simulink model "MOBATSim_AutoTesting"  (R2020b)
settings: Solver=VariableStepAuto  StartTime=0.0  StopTime=20  FixedStep=0.01  RelTol=1e-3
undefined symbols (not defined in the file or in its folder): default_spacing, FI_distance, FI_speed, max_ac, meters, min_ac, SafeDistance, Sim_Ts, simSpeed, time_gap, Ts, v_set, Vehicle1, Vehicle10, Vehicle2, Vehicle3, Vehicle4, Vehicle5, Vehicle6, Vehicle7, Vehicle8, Vehicle9, verr_gain, vx_gain, xerr_gain
libraries: simulink x21, pid_lib x11, mpcadaslib x1
(part 1 of 4)
settings Model: Creator=Mustafa  LastModifiedBy=62783
settings SolverCC: AutoInsertRateTranBlk=on  InsertRTBMode=Always  MinimalZcImpactIntegration=on
settings DataIOCC: ReturnWorkspaceOutputs=off
settings DebuggingCC: AlgebraicLoopMsg=error  ArithmeticOperatorsInVariantConditions=warning
settings SFSimCC: SimUseLocalCustomCode=off  CustomCodeUndefinedFunction=UseInterfaceOnly
settings RTWCC: RTWUseLocalCustomCode=off
settings CodeAppCC: StateflowObjectComments=on

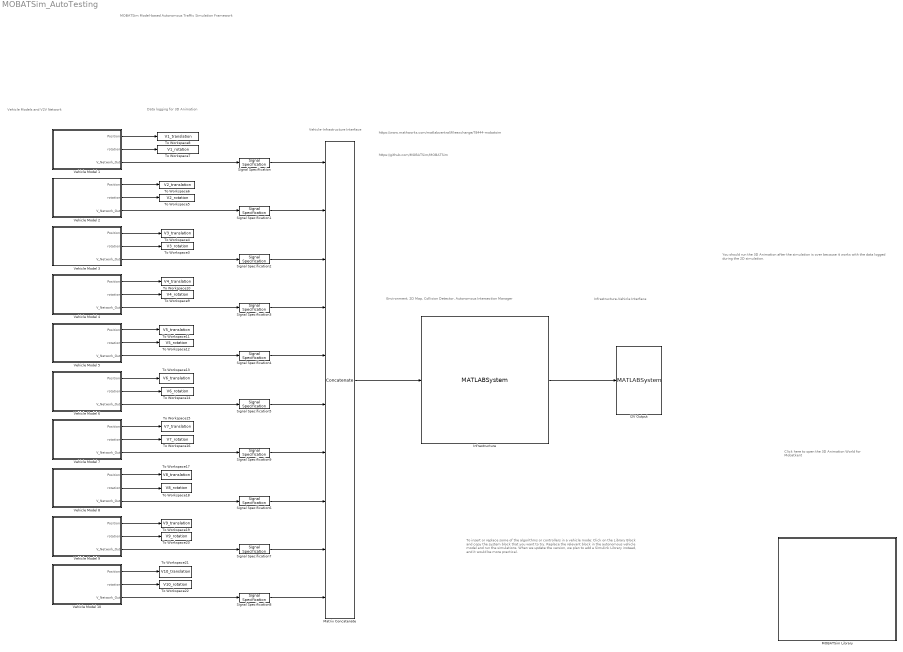
== system MOBATSim_AutoTesting ==
  note: https://www.mathworks.com/matlabcentral/fileexchange/78444-mobatsim
  note: https://github.com/MOBATSim/MOBATSim
  note: To insert or replace some of the algorithms
      | or controllers in a vehicle mode:
      | Click on the Library Block and copy the system block that you want to try.
      | Replace the relevant block in the autonomous vehicle model and run the simulations.
      | When we update the version, we plan to add a Simulink Library instead, and it would be more practical.
  note: MOBATSim
      | Model-based Autonomous Traffic Simulation Framework
  note: You should run the 3D Animation after the simulation is over because it works with the data logged during the 2D simulation.
  note: Click here to open the 3D Animation World for Mobatkent
  note: Infrastructure-Vehicle Interface
  note: Data logging for 3D Animation
  note: Vehicle Models and V2V Network
  note: Environment, 2D Map, Collision Detector, Autonomous Intersection Manager
  note: Vehicle-Infrastructure Interface
  I2V Output : MATLABSystem  System=I2V  SimulateUsing=Interpreted execution
      mask Type: I2V
      mask Display:
      | image('I2V.png');
      | port_label('input',1,'Flags');
  Infrastructure : MATLABSystem  Description=An instance of the Map.m Class is created.  System=Infrastructure  SimulateUsing=Interpreted execution
      mask Type: Infrastructure
      mask Display:
      | image('logo_small.png');
      | port_label('input',1,'V2Idata');
      | port_label('output',1,'mergedBrakingFlagArrays');
  MOBATSim Library : Subsystem
      mask Display: image('$imagefile'); % Use "Edit Image" on toolstrip to change.
  Matrix Concatenate : Concatenate  NumInputs=10  Mode=Multidimensional array
  Signal Specification{,1..9} (10 alike) : SignalSpecification  Dimensions=[1 2]
  To Workspace10 : ToWorkspace  VariableName=V4_translation  SaveFormat=Timeseries  SampleTime=-1
  To Workspace11 : ToWorkspace  VariableName=V5_translation  SaveFormat=Timeseries  SampleTime=-1
  To Workspace12 : ToWorkspace  VariableName=V5_rotation  SaveFormat=Timeseries  SampleTime=-1
  To Workspace13 : ToWorkspace  VariableName=V6_translation  SaveFormat=Timeseries  SampleTime=-1
  To Workspace14 : ToWorkspace  VariableName=V6_rotation  SaveFormat=Timeseries  SampleTime=-1
  To Workspace15 : ToWorkspace  VariableName=V7_translation  SaveFormat=Timeseries  SampleTime=-1
  To Workspace16 : ToWorkspace  VariableName=V7_rotation  SaveFormat=Timeseries  SampleTime=-1
  To Workspace17 : ToWorkspace  VariableName=V8_translation  SaveFormat=Timeseries  SampleTime=-1
  To Workspace18 : ToWorkspace  VariableName=V8_rotation  SaveFormat=Timeseries  SampleTime=-1
  To Workspace19 : ToWorkspace  VariableName=V9_translation  SaveFormat=Timeseries  SampleTime=-1
  To Workspace20 : ToWorkspace  VariableName=V9_rotation  SaveFormat=Timeseries  SampleTime=-1
  To Workspace21 : ToWorkspace  VariableName=V10_translation  SaveFormat=Timeseries  SampleTime=-1
  To Workspace22 : ToWorkspace  VariableName=V10_rotation  SaveFormat=Timeseries  SampleTime=-1
  To Workspace3 : ToWorkspace  VariableName=V3_rotation  SaveFormat=Timeseries  SampleTime=-1
  To Workspace4 : ToWorkspace  VariableName=V3_translation  SaveFormat=Timeseries  SampleTime=-1
  To Workspace5 : ToWorkspace  VariableName=V2_rotation  SaveFormat=Timeseries  SampleTime=-1
  To Workspace6 : ToWorkspace  VariableName=V2_translation  SaveFormat=Timeseries  SampleTime=-1
  To Workspace7 : ToWorkspace  VariableName=V1_rotation  SaveFormat=Timeseries  SampleTime=-1
  To Workspace8 : ToWorkspace  VariableName=V1_translation  SaveFormat=Timeseries  SampleTime=-1
  To Workspace9 : ToWorkspace  VariableName=V4_rotation  SaveFormat=Timeseries  SampleTime=-1
  Vehicle Model 1 : Subsystem  Description=Tag: Autonomous Vehicle Model  SystemSampleTime=0.01  mask{Pos=Vehicle1.dynamics.position, Vehicle_id=[1], SpeedScale=1/simSpeed, maxSpeed=Vehicle1.dynamics.maxSpeed, MinDeceleration=Vehicle1.dynamics.minDeceleration, FI_distance=FI_distance, FI_speed=FI_speed, meters=SafeDistance}
      mask prompts: Pos "Initial Position"; FI_distance "FI_Distance_Sensor"; meters "SafeDistance"
      mask TypeOptions Pos: initial position/Value
      mask TypeOptions Vehicle_id: MATLAB System2/Vehicle_id
      mask TypeOptions SpeedScale: scale the movement/Gain
      mask TypeOptions maxSpeed: Longitudinal Speed Control/Platoon Controller/Saturation3/UpperLimit
      mask TypeOptions MinDeceleration: Longitudinal Speed Control/Acceleration Command/Emergency Brake/Value
      mask TypeOptions FI_distance: Fault Injection Percentage/Value
      mask TypeOptions FI_speed: Longitudinal Speed Control/FI Freeze/Constant/Value
      mask TypeOptions meters: Longitudinal Speed Control/Platoon Controller/Constant/Value
      mask DialogControl DescTextVar Prompt: Autonomous Vehicle Model defined as a system, press the arrow on the lower left corner to see the subsystems. The initial parameters below should be taken from the base workspace but you can edit them anyway you like.
      mask Display: image('$imagefile'); % Use "Edit Image" on toolstrip to change.
  Vehicle Model 10 : Subsystem  Description=Tag: Autonomous Vehicle Model  SystemSampleTime=0.01  mask{Pos=Vehicle10.dynamics.position, Vehicle_id=[10], SpeedScale=1/simSpeed, maxSpeed=Vehicle10.dynamics.maxSpeed, MinDeceleration=Vehicle10.dynamics.minDeceleration, FI_distance=FI_distance, FI_speed=FI_speed, meters=SafeDistance}
      mask prompts: Pos "Initial Position"; FI_distance "FI_Distance_Sensor"; meters "SafeDistance"
      mask TypeOptions Pos: initial position/Value
      mask TypeOptions Vehicle_id: MATLAB System2/Vehicle_id
      mask TypeOptions SpeedScale: scale the movement/Gain
      mask TypeOptions maxSpeed: Longitudinal Speed Control/Platoon Controller/Saturation3/UpperLimit
      mask TypeOptions MinDeceleration: Longitudinal Speed Control/Acceleration Command/Emergency Brake/Value
      mask TypeOptions FI_distance: Fault Injection Percentage/Value
      mask TypeOptions FI_speed: Longitudinal Speed Control/FI Freeze/Constant/Value
      mask TypeOptions meters: Longitudinal Speed Control/Platoon Controller/Constant/Value
      mask DialogControl DescTextVar Prompt: Autonomous Vehicle Model defined as a system, press the arrow on the lower left corner to see the subsystems. The initial parameters below should be taken from the base workspace but you can edit them anyway you like.
      mask Display: image('redcar.png'); % Use "Edit Image" on toolstrip to change.
  Vehicle Model 2 : Subsystem  Description=Tag: Autonomous Vehicle Model  SystemSampleTime=0.01  mask{Pos=Vehicle2.dynamics.position, Vehicle_id=[2], SpeedScale=1/simSpeed, maxSpeed=Vehicle2.dynamics.maxSpeed, MinDeceleration=Vehicle2.dynamics.minDeceleration, FI_distance=FI_distance, FI_speed=FI_speed, meters=SafeDistance}
      mask prompts: Pos "Initial Position"; FI_distance "FI_Distance_Sensor"; meters "SafeDistance"
      mask TypeOptions Pos: initial position/Value
      mask TypeOptions Vehicle_id: MATLAB System2/Vehicle_id
      mask TypeOptions SpeedScale: scale the movement/Gain
      mask TypeOptions maxSpeed: Longitudinal Speed Control/Platoon Controller/Saturation3/UpperLimit
      mask TypeOptions MinDeceleration: Longitudinal Speed Control/Acceleration Command/Emergency Brake/Value
      mask TypeOptions FI_distance: Fault Injection Percentage/Value
      mask TypeOptions FI_speed: Longitudinal Speed Control/FI Freeze/Constant/Value
      mask TypeOptions meters: Longitudinal Speed Control/Platoon Controller/Constant/Value
      mask DialogControl DescTextVar Prompt: Autonomous Vehicle Model defined as a system, press the arrow on the lower left corner to see the subsystems. The initial parameters below should be taken from the base workspace but you can edit them anyway you like.
      mask Display: image('$imagefile'); % Use "Edit Image" on toolstrip to change.
  Vehicle Model 3 : Subsystem  Description=Tag: Autonomous Vehicle Model  SystemSampleTime=0.01  mask{Pos=Vehicle3.dynamics.position, Vehicle_id=[3], SpeedScale=1/simSpeed, maxSpeed=Vehicle3.dynamics.maxSpeed, MinDeceleration=Vehicle3.dynamics.minDeceleration, FI_distance=FI_distance, FI_speed=FI_speed, meters=SafeDistance}
      mask prompts: Pos "Initial Position"; FI_distance "FI_Distance_Sensor"; meters "SafeDistance"
      mask TypeOptions Pos: initial position/Value
      mask TypeOptions Vehicle_id: MATLAB System2/Vehicle_id
      mask TypeOptions SpeedScale: scale the movement/Gain
      mask TypeOptions maxSpeed: Longitudinal Speed Control/Platoon Controller/Saturation3/UpperLimit
      mask TypeOptions MinDeceleration: Longitudinal Speed Control/Acceleration Command/Emergency Brake/Value
      mask TypeOptions FI_distance: Fault Injection Percentage/Value
      mask TypeOptions FI_speed: Longitudinal Speed Control/FI Freeze/Constant/Value
      mask TypeOptions meters: Longitudinal Speed Control/Platoon Controller/Constant/Value
      mask DialogControl DescTextVar Prompt: Autonomous Vehicle Model defined as a system, press the arrow on the lower left corner to see the subsystems. The initial parameters below should be taken from the base workspace but you can edit them anyway you like.
      mask Display: image('$imagefile'); % Use "Edit Image" on toolstrip to change.
  Vehicle Model 4 : Subsystem  Description=Tag: Autonomous Vehicle Model  SystemSampleTime=0.01  mask{Pos=Vehicle4.dynamics.position, Vehicle_id=[4], SpeedScale=1/simSpeed, maxSpeed=Vehicle4.dynamics.maxSpeed, MinDeceleration=Vehicle4.dynamics.minDeceleration, FI_distance=FI_distance, FI_speed=FI_speed, meters=SafeDistance}
      mask prompts: Pos "Initial Position"; FI_distance "FI_Distance_Sensor"; meters "SafeDistance"
      mask TypeOptions Pos: initial position/Value
      mask TypeOptions Vehicle_id: MATLAB System2/Vehicle_id
      mask TypeOptions SpeedScale: scale the movement/Gain
      mask TypeOptions maxSpeed: Longitudinal Speed Control/Platoon Controller/Saturation3/UpperLimit
      mask TypeOptions MinDeceleration: Longitudinal Speed Control/Acceleration Command/Emergency Brake/Value
      mask TypeOptions FI_distance: Fault Injection Percentage/Value
      mask TypeOptions FI_speed: Longitudinal Speed Control/FI Freeze/Constant/Value
      mask TypeOptions meters: Longitudinal Speed Control/Platoon Controller/Constant/Value
      mask DialogControl DescTextVar Prompt: Autonomous Vehicle Model defined as a system, press the arrow on the lower left corner to see the subsystems. The initial parameters below should be taken from the base workspace but you can edit them anyway you like.
      mask Display: image('$imagefile'); % Use "Edit Image" on toolstrip to change.
  Vehicle Model 5 : Subsystem  Description=Tag: Autonomous Vehicle Model  SystemSampleTime=0.01  mask{Pos=Vehicle5.dynamics.position, Vehicle_id=[5], SpeedScale=1/simSpeed, maxSpeed=Vehicle5.dynamics.maxSpeed, MinDeceleration=Vehicle5.dynamics.minDeceleration, FI_distance=FI_distance, FI_speed=FI_speed, meters=SafeDistance}
      mask prompts: Pos "Initial Position"; FI_distance "FI_Distance_Sensor"; meters "SafeDistance"
      mask TypeOptions Pos: initial position/Value
      mask TypeOptions Vehicle_id: MATLAB System2/Vehicle_id
      mask TypeOptions SpeedScale: scale the movement/Gain
      mask TypeOptions maxSpeed: Longitudinal Speed Control/Platoon Controller/Saturation3/UpperLimit
      mask TypeOptions MinDeceleration: Longitudinal Speed Control/Acceleration Command/Emergency Brake/Value
      mask TypeOptions FI_distance: Fault Injection Percentage/Value
      mask TypeOptions FI_speed: Longitudinal Speed Control/FI Freeze/Constant/Value
      mask TypeOptions meters: Longitudinal Speed Control/Platoon Controller/Constant/Value
      mask DialogControl DescTextVar Prompt: Autonomous Vehicle Model defined as a system, press the arrow on the lower left corner to see the subsystems. The initial parameters below should be taken from the base workspace but you can edit them anyway you like.
      mask Display: image('$imagefile'); % Use "Edit Image" on toolstrip to change.
  Vehicle Model 6 : Subsystem  Description=Tag: Autonomous Vehicle Model  SystemSampleTime=0.01  mask{Pos=Vehicle6.dynamics.position, Vehicle_id=[6], SpeedScale=1/simSpeed, maxSpeed=Vehicle6.dynamics.maxSpeed, MinDeceleration=Vehicle6.dynamics.minDeceleration, FI_distance=FI_distance, FI_speed=FI_speed, meters=SafeDistance}
      mask prompts: Pos "Initial Position"; FI_distance "FI_Distance_Sensor"; meters "SafeDistance"
      mask TypeOptions Pos: initial position/Value
      mask TypeOptions Vehicle_id: MATLAB System2/Vehicle_id
      mask TypeOptions SpeedScale: scale the movement/Gain
      mask TypeOptions maxSpeed: Longitudinal Speed Control/Platoon Controller/Saturation3/UpperLimit
      mask TypeOptions MinDeceleration: Longitudinal Speed Control/Acceleration Command/Emergency Brake/Value
      mask TypeOptions FI_distance: Fault Injection Percentage/Value
      mask TypeOptions FI_speed: Longitudinal Speed Control/FI Freeze/Constant/Value
      mask TypeOptions meters: Longitudinal Speed Control/Platoon Controller/Constant/Value
      mask DialogControl DescTextVar Prompt: Autonomous Vehicle Model defined as a system, press the arrow on the lower left corner to see the subsystems. The initial parameters below should be taken from the base workspace but you can edit them anyway you like.
      mask Display: image('firetruck.png'); % Use "Edit Image" on toolstrip to change.
  Vehicle Model 7 : Subsystem  Description=Tag: Autonomous Vehicle Model  SystemSampleTime=0.01  mask{Pos=Vehicle7.dynamics.position, Vehicle_id=[7], SpeedScale=1/simSpeed, maxSpeed=Vehicle7.dynamics.maxSpeed, MinDeceleration=Vehicle7.dynamics.minDeceleration, FI_distance=FI_distance, FI_speed=FI_speed, meters=SafeDistance}
      mask prompts: Pos "Initial Position"; FI_distance "FI_Distance_Sensor"; meters "SafeDistance"
      mask TypeOptions Pos: initial position/Value
      mask TypeOptions Vehicle_id: MATLAB System2/Vehicle_id
      mask TypeOptions SpeedScale: scale the movement/Gain
      mask TypeOptions maxSpeed: Longitudinal Speed Control/Platoon Controller/Saturation3/UpperLimit
      mask TypeOptions MinDeceleration: Longitudinal Speed Control/Acceleration Command/Emergency Brake/Value
      mask TypeOptions FI_distance: Fault Injection Percentage/Value
      mask TypeOptions FI_speed: Longitudinal Speed Control/FI Freeze/Constant/Value
      mask TypeOptions meters: Longitudinal Speed Control/Platoon Controller/Constant/Value
      mask DialogControl DescTextVar Prompt: Autonomous Vehicle Model defined as a system, press the arrow on the lower left corner to see the subsystems. The initial parameters below should be taken from the base workspace but you can edit them anyway you like.
      mask Display: image('$imagefile'); % Use "Edit Image" on toolstrip to change.
  Vehicle Model 8 : Subsystem  Description=Tag: Autonomous Vehicle Model  SystemSampleTime=0.01  mask{Pos=Vehicle8.dynamics.position, Vehicle_id=[8], SpeedScale=1/simSpeed, maxSpeed=Vehicle8.dynamics.maxSpeed, MinDeceleration=Vehicle8.dynamics.minDeceleration, FI_distance=FI_distance, FI_speed=FI_speed, meters=SafeDistance}
      mask prompts: Pos "Initial Position"; FI_distance "FI_Distance_Sensor"; meters "SafeDistance"
      mask TypeOptions Pos: initial position/Value
      mask TypeOptions Vehicle_id: MATLAB System2/Vehicle_id
      mask TypeOptions SpeedScale: scale the movement/Gain
      mask TypeOptions maxSpeed: Longitudinal Speed Control/Platoon Controller/Saturation3/UpperLimit
      mask TypeOptions MinDeceleration: Longitudinal Speed Control/Acceleration Command/Emergency Brake/Value
      mask TypeOptions FI_distance: Fault Injection Percentage/Value
      mask TypeOptions FI_speed: Longitudinal Speed Control/FI Freeze/Constant/Value
      mask TypeOptions meters: Longitudinal Speed Control/Platoon Controller/Constant/Value
      mask DialogControl DescTextVar Prompt: Autonomous Vehicle Model defined as a system, press the arrow on the lower left corner to see the subsystems. The initial parameters below should be taken from the base workspace but you can edit them anyway you like.
      mask Display: image('$imagefile'); % Use "Edit Image" on toolstrip to change.
  Vehicle Model 9 : Subsystem  Description=Tag: Autonomous Vehicle Model  SystemSampleTime=0.01  mask{Pos=Vehicle9.dynamics.position, Vehicle_id=[9], SpeedScale=1/simSpeed, maxSpeed=Vehicle9.dynamics.maxSpeed, MinDeceleration=Vehicle9.dynamics.minDeceleration, FI_distance=FI_distance, FI_speed=FI_speed, meters=SafeDistance}
      mask prompts: Pos "Initial Position"; FI_distance "FI_Distance_Sensor"; meters "SafeDistance"
      mask TypeOptions Pos: initial position/Value
      mask TypeOptions Vehicle_id: MATLAB System2/Vehicle_id
      mask TypeOptions SpeedScale: scale the movement/Gain
      mask TypeOptions maxSpeed: Longitudinal Speed Control/Platoon Controller/Saturation3/UpperLimit
      mask TypeOptions MinDeceleration: Longitudinal Speed Control/Acceleration Command/Emergency Brake/Value
      mask TypeOptions FI_distance: Fault Injection Percentage/Value
      mask TypeOptions FI_speed: Longitudinal Speed Control/FI Freeze/Constant/Value
      mask TypeOptions meters: Longitudinal Speed Control/Platoon Controller/Constant/Value
      mask DialogControl DescTextVar Prompt: Autonomous Vehicle Model defined as a system, press the arrow on the lower left corner to see the subsystems. The initial parameters below should be taken from the base workspace but you can edit them anyway you like.
      mask Display: image('$imagefile'); % Use "Edit Image" on toolstrip to change.
  wires:
  Vehicle Model 1/1(Position) -> To Workspace8/1
  Vehicle Model 1/2(rotation) -> To Workspace7/1
  Vehicle Model 1/3(V_Network_Out) -> Signal Specification/1
  Signal Specification/1 -> Matrix Concatenate/1
  Signal Specification1/1 -> Matrix Concatenate/2
  Vehicle Model 2/2(rotation) -> To Workspace5/1
  Vehicle Model 2/1(Position) -> To Workspace6/1
  Vehicle Model 3/2(rotation) -> To Workspace3/1
  Vehicle Model 3/1(Position) -> To Workspace4/1
  Signal Specification2/1 -> Matrix Concatenate/3
  Infrastructure/1 -> I2V Output/1
  Vehicle Model 8/3(V_Network_Out) -> Signal Specification6/1
  Vehicle Model 9/3(V_Network_Out) -> Signal Specification7/1
  Vehicle Model 10/3(V_Network_Out) -> Signal Specification8/1
  Signal Specification3/1 -> Matrix Concatenate/4
  Signal Specification4/1 -> Matrix Concatenate/5
  Signal Specification5/1 -> Matrix Concatenate/6
  Signal Specification9/1 -> Matrix Concatenate/7
  Signal Specification6/1 -> Matrix Concatenate/8
  Signal Specification7/1 -> Matrix Concatenate/9
  Signal Specification8/1 -> Matrix Concatenate/10
  Vehicle Model 4/2(rotation) -> To Workspace9/1
  Vehicle Model 4/1(Position) -> To Workspace10/1
  Vehicle Model 5/1(Position) -> To Workspace11/1
  Vehicle Model 5/2(rotation) -> To Workspace12/1
  Vehicle Model 6/2(rotation) -> To Workspace14/1
  Vehicle Model 6/1(Position) -> To Workspace13/1
  Vehicle Model 7/2(rotation) -> To Workspace16/1
  Vehicle Model 7/1(Position) -> To Workspace15/1
  Vehicle Model 8/2(rotation) -> To Workspace18/1
  Vehicle Model 8/1(Position) -> To Workspace17/1
  Vehicle Model 9/2(rotation) -> To Workspace20/1
  Vehicle Model 9/1(Position) -> To Workspace19/1
  Vehicle Model 10/2(rotation) -> To Workspace22/1
  Vehicle Model 10/1(Position) -> To Workspace21/1
  Matrix Concatenate/1 -> Infrastructure/1
  Vehicle Model 2/3(V_Network_Out) -> Signal Specification1/1
  Vehicle Model 3/3(V_Network_Out) -> Signal Specification2/1
  Vehicle Model 4/3(V_Network_Out) -> Signal Specification3/1
  Vehicle Model 5/3(V_Network_Out) -> Signal Specification4/1
  Vehicle Model 6/3(V_Network_Out) -> Signal Specification5/1
  Vehicle Model 7/3(V_Network_Out) -> Signal Specification9/1

== system MOBATSim_AutoTesting/MOBATSim Library ==
  note: Different pathplanner algorithms with the same input/outputs. Some details and computational performances may differ.
  note: The ACC Classical Block from the MathWorks Example:
      | https://www.mathworks.com/help/driving/examples/adaptive-cruise-control-with-sensor-fusion.html
  note: Path Planners - MATLAB System Blocks
  note: Platoon Controllers - Subsystem Blocks
  note: Platoon controller-PID with a safe distance controller for safely following the
      | leading vehicle. Most vehicles have this block because it is simple and fast
      | in terms of execution time. Can be tuned.
  note: Standard MPC - Adaptive Cruise Control Block. Safest option but computationally
      | expensive. Tradeoff between safety and computational performance depends on
      | the prediction horizon variable.
  ACC Classical : Subsystem  Commented=on  TreatAsAtomicUnit=on  VariantControl=controller_type == 1
      settings: RTWFileNameOpts=Use function name
  Adaptive Cruise Control System : mpcadaslib/Adaptive Cruise Control System  Commented=on  EgoModel=tf(1,[0.5,1,0])  InitialEgoVelocity=20  DefaultSpacing=10  MaxVelocity=50  MinAcceleration=-3  amin_ext=off  MaxAcceleration=2  amax_ext=off  Ts=0.1  PredictionHorizon=30  ControllerBehavior=0.5  suboptimal=off  maxiter=10  datatypeopt=double  optmode=off  trackmode=off
  Path Planner - AStar : MATLABSystem  Commented=on  System=VehiclePathPlanner  Vehicle_id=[]  SimulateUsing=Code generation
      mask Type: VehiclePathPlanner
      mask Display:
      | disp('VehiclePathPlanner');
      | port_label('input',1,'OtherVehiclesFutureData');
      | port_label('output',1,'FuturePlan');
      | port_label('output',2,'waypointReached');
  Path Planner - DStar : MATLABSystem  Commented=on  System=VehiclePathPlanner_DStarExtraLight  Vehicle_id=[]  SimulateUsing=Code generation
      mask Type: VehiclePathPlanner_DStarExtraLight
      mask Display:
      | disp('VehiclePathPlanner_DStarExtraLight');
      | port_label('input',1,'OtherVehiclesFutureData');
      | port_label('output',1,'FuturePlan');
      | port_label('output',2,'waypointReached');
  Path Planner - Shortest : MATLABSystem  Commented=on  System=VehiclePathPlanner_shortestPathFinder  Vehicle_id=[]  SimulateUsing=Code generation
      mask Type: VehiclePathPlanner_shortestPathFinder
      mask Display:
      | disp('VehiclePathPlanner_shortestPathFinder');
      | port_label('input',1,'OtherVehiclesFutureData');
      | port_label('output',1,'FuturePlan');
      | port_label('output',2,'waypointReached');
  Platoon Controller - PID : Subsystem  Commented=on

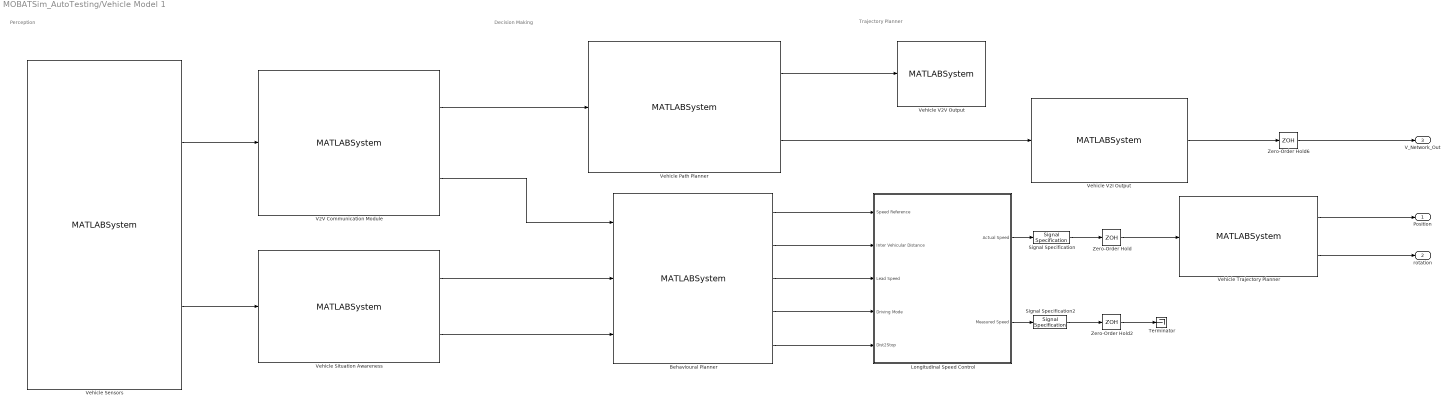
== system MOBATSim_AutoTesting/Vehicle Model 1 ==
  note: Trajectory Planner
  note: Perception
  note: Decision Making
  Behavioural Planner : MATLABSystem  System=VehicleDrivingMode  Vehicle_id=Vehicle_id  SimulateUsing=Interpreted execution
      mask Type: VehicleDrivingMode
      mask Display:
      | image('BehaviouralPlanner.png');
      | port_label('input',1,'LeaderSpeed');
      | port_label('input',2,'LeaderDistance');
      | port_label('input',3,'emergencyCase');
      | port_label('output',1,'SpeedReference');
      | port_label('output',2,'DistanceReference');
      | port_label('output',3,'LeadSpeed');
      | port_label('output',4,'DrivingMode');
      | port_label('output',5,'Dist2Stop');
  Longitudinal Speed Control : Subsystem
  Signal Specification : SignalSpecification  Dimensions=1
  Signal Specification2 : SignalSpecification  Dimensions=1
  Terminator : Terminator
  V2V Communication Module : MATLABSystem  System=VehicleCommunication_v2v  Vehicle_id=Vehicle_id  SimulateUsing=Interpreted execution
      mask Type: VehicleCommunication_v2v
      mask Display:
      | image('V2V.png');
      | port_label('input',1,'CommunicationID');
      | port_label('output',1,'OtherVehiclesFutureData');
      | port_label('output',2,'LeaderSpeed');
  Vehicle Path Planner : MATLABSystem  System=VehiclePathPlanner  Vehicle_id=Vehicle_id  SimulateUsing=Interpreted execution
      mask Type: VehiclePathPlanner
      mask Display:
      | image('PathPlanner.png');
      | port_label('input',1,'OtherVehiclesFutureData');
      | port_label('output',1,'FuturePlan');
      | port_label('output',2,'waypointReached');
  Vehicle Sensors : MATLABSystem  System=VehicleSensors  Vehicle_id=Vehicle_id  Tsample=Sim_Ts  OffsetTime=0  SimulateUsing=Interpreted execution
      mask Type: VehicleSensors
      mask Display:
      | image('sensor.png');
      | port_label('output',1,'V2VcommIDs');
      | port_label('output',2,'ObjectinFront');
  Vehicle Situation Awareness : MATLABSystem  System=VehicleSituationAwareness  Vehicle_id=Vehicle_id  SimulateUsing=Interpreted execution
      mask Type: VehicleSituationAwareness
      mask Display:
      | image('situationAwareness.png');
      | port_label('input',1,'FrontSensorData');
      | port_label('output',1,'leaderDistance');
      | port_label('output',2,'emergencyCase');
  Vehicle Trajectory Planner : MATLABSystem  System=VehicleKinematics  Vehicle_id=Vehicle_id  SimulateUsing=Interpreted execution
      mask Type: VehicleKinematics
      mask Display:
      | image('Vehicle.png');
      | port_label('input',1,'speed');
      | port_label('output',1,'position');
      | port_label('output',2,'rotation');
  Vehicle V2I Output : MATLABSystem  System=VehicleV2I_Out  Vehicle_id=Vehicle_id  SimulateUsing=Interpreted execution
      mask Type: VehicleV2I_Out
      mask Display:
      | image('V2I.png');
      | port_label('input',1,'waypointReached');
      | port_label('output',1,'V2Idata');
  Vehicle V2V Output : MATLABSystem  System=VehicleNetwork_Out  Vehicle_id=Vehicle_id  SimulateUsing=Interpreted execution
      mask Type: VehicleNetwork_Out
      mask Display:
      | image('V2V.png');
      | port_label('input',1,'FuturePlan');
  Zero-Order Hold : ZeroOrderHold  SampleTime=Sim_Ts
  Zero-Order Hold2 : ZeroOrderHold  SampleTime=Sim_Ts
  Zero-Order Hold6 : ZeroOrderHold  SampleTime=Sim_Ts
  Position : Outport  VectorParamsAs1DForOutWhenUnconnected=off
  rotation : Outport  Port=2  VectorParamsAs1DForOutWhenUnconnected=off
  V_Network_Out : Outport  Port=3  VectorParamsAs1DForOutWhenUnconnected=off
  wires:
  Vehicle Trajectory Planner/1 -> Position/1
  Vehicle Trajectory Planner/2 -> rotation/1
  Signal Specification/1 -> Zero-Order Hold/1
  Zero-Order Hold/1 -> Vehicle Trajectory Planner/1
  Signal Specification2/1 -> Zero-Order Hold2/1
  Longitudinal Speed Control/1(Actual Speed) -> Signal Specification/1
  Vehicle V2I Output/1 -> Zero-Order Hold6/1
  Longitudinal Speed Control/2(Measured Speed) -> Signal Specification2/1
  Zero-Order Hold2/1 -> Terminator/1
  Vehicle Sensors/2 -> Vehicle Situation Awareness/1
  Vehicle Situation Awareness/2 -> Behavioural Planner/3
  Vehicle Situation Awareness/1 -> Behavioural Planner/2
  V2V Communication Module/2 -> Behavioural Planner/1
  V2V Communication Module/1 -> Vehicle Path Planner/1
  Behavioural Planner/5 -> Longitudinal Speed Control/5(Dist2Stop)
  Behavioural Planner/4 -> Longitudinal Speed Control/4(Driving Mode)
  Behavioural Planner/3 -> Longitudinal Speed Control/3(Lead Speed)
  Behavioural Planner/2 -> Longitudinal Speed Control/2(Inter Vehicular Distance)
  Behavioural Planner/1 -> Longitudinal Speed Control/1(Speed Reference)
  Vehicle Path Planner/2 -> Vehicle V2I Output/1
  Vehicle Path Planner/1 -> Vehicle V2V Output/1
  Vehicle Sensors/1 -> V2V Communication Module/1
  Zero-Order Hold6/1 -> V_Network_Out/1

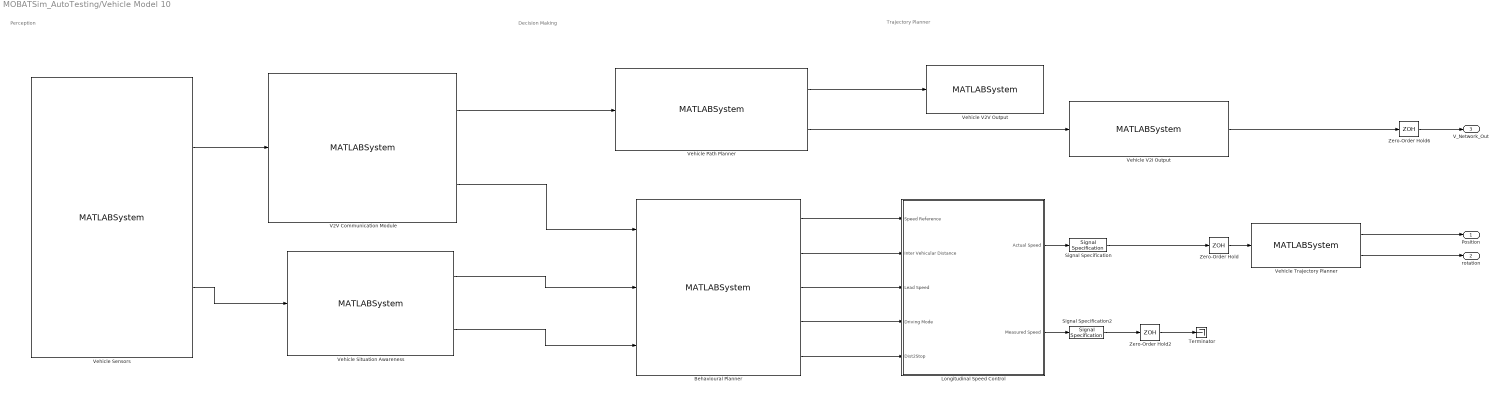
== system MOBATSim_AutoTesting/Vehicle Model 10 ==
  note: Trajectory Planner
  note: Perception
  note: Decision Making
  Behavioural Planner : MATLABSystem  System=VehicleDrivingMode  Vehicle_id=Vehicle_id  SimulateUsing=Interpreted execution
      mask Type: VehicleDrivingMode
      mask Display:
      | image('BehaviouralPlanner.png');
      | port_label('input',1,'LeaderSpeed');
      | port_label('input',2,'LeaderDistance');
      | port_label('input',3,'emergencyCase');
      | port_label('output',1,'SpeedReference');
      | port_label('output',2,'DistanceReference');
      | port_label('output',3,'LeadSpeed');
      | port_label('output',4,'DrivingMode');
      | port_label('output',5,'Dist2Stop');
  Longitudinal Speed Control : Subsystem
  Signal Specification : SignalSpecification  Dimensions=1
  Signal Specification2 : SignalSpecification  Dimensions=1
  Terminator : Terminator
  V2V Communication Module : MATLABSystem  System=VehicleCommunication_v2v  Vehicle_id=Vehicle_id  SimulateUsing=Interpreted execution
      mask Type: VehicleCommunication_v2v
      mask Display:
      | image('V2V.png');
      | port_label('input',1,'CommunicationID');
      | port_label('output',1,'OtherVehiclesFutureData');
      | port_label('output',2,'LeaderSpeed');
  Vehicle Path Planner : MATLABSystem  System=VehiclePathPlanner  Vehicle_id=Vehicle_id  SimulateUsing=Interpreted execution
      mask Type: VehiclePathPlanner
      mask Display:
      | image('PathPlanner.png');
      | port_label('input',1,'OtherVehiclesFutureData');
      | port_label('output',1,'FuturePlan');
      | port_label('output',2,'waypointReached');
  Vehicle Sensors : MATLABSystem  System=VehicleSensors  Vehicle_id=Vehicle_id  Tsample=Sim_Ts  OffsetTime=0  SimulateUsing=Interpreted execution
      mask Type: VehicleSensors
      mask Display:
      | image('sensor.png');
      | port_label('output',1,'V2VcommIDs');
      | port_label('output',2,'ObjectinFront');
  Vehicle Situation Awareness : MATLABSystem  System=VehicleSituationAwareness  Vehicle_id=Vehicle_id  SimulateUsing=Interpreted execution
      mask Type: VehicleSituationAwareness
      mask Display:
      | image('situationAwareness.png');
      | port_label('input',1,'FrontSensorData');
      | port_label('output',1,'leaderDistance');
      | port_label('output',2,'emergencyCase');
  Vehicle Trajectory Planner : MATLABSystem  System=VehicleKinematics  Vehicle_id=Vehicle_id  SimulateUsing=Interpreted execution
      mask Type: VehicleKinematics
      mask Display:
      | image('Vehicle.png');
      | port_label('input',1,'speed');
      | port_label('output',1,'position');
      | port_label('output',2,'rotation');
  Vehicle V2I Output : MATLABSystem  System=VehicleV2I_Out  Vehicle_id=Vehicle_id  SimulateUsing=Interpreted execution
      mask Type: VehicleV2I_Out
      mask Display:
      | image('V2I.png');
      | port_label('input',1,'waypointReached');
      | port_label('output',1,'V2Idata');
  Vehicle V2V Output : MATLABSystem  System=VehicleNetwork_Out  Vehicle_id=Vehicle_id  SimulateUsing=Interpreted execution
      mask Type: VehicleNetwork_Out
      mask Display:
      | image('V2V.png');
      | port_label('input',1,'FuturePlan');
  Zero-Order Hold : ZeroOrderHold  SampleTime=Sim_Ts
  Zero-Order Hold2 : ZeroOrderHold  SampleTime=Sim_Ts
  Zero-Order Hold6 : ZeroOrderHold  SampleTime=Sim_Ts
  Position : Outport  VectorParamsAs1DForOutWhenUnconnected=off
  rotation : Outport  Port=2  VectorParamsAs1DForOutWhenUnconnected=off
  V_Network_Out : Outport  Port=3  VectorParamsAs1DForOutWhenUnconnected=off
  wires:
  Vehicle Trajectory Planner/1 -> Position/1
  Vehicle Trajectory Planner/2 -> rotation/1
  Signal Specification/1 -> Zero-Order Hold/1
  Zero-Order Hold/1 -> Vehicle Trajectory Planner/1
  Signal Specification2/1 -> Zero-Order Hold2/1
  Longitudinal Speed Control/1(Actual Speed) -> Signal Specification/1
  Vehicle V2I Output/1 -> Zero-Order Hold6/1
  Longitudinal Speed Control/2(Measured Speed) -> Signal Specification2/1
  Zero-Order Hold2/1 -> Terminator/1
  Vehicle Sensors/2 -> Vehicle Situation Awareness/1
  Vehicle Situation Awareness/2 -> Behavioural Planner/3
  Vehicle Situation Awareness/1 -> Behavioural Planner/2
  V2V Communication Module/2 -> Behavioural Planner/1
  V2V Communication Module/1 -> Vehicle Path Planner/1
  Behavioural Planner/5 -> Longitudinal Speed Control/5(Dist2Stop)
  Behavioural Planner/4 -> Longitudinal Speed Control/4(Driving Mode)
  Behavioural Planner/3 -> Longitudinal Speed Control/3(Lead Speed)
  Behavioural Planner/2 -> Longitudinal Speed Control/2(Inter Vehicular Distance)
  Behavioural Planner/1 -> Longitudinal Speed Control/1(Speed Reference)
  Vehicle Path Planner/2 -> Vehicle V2I Output/1
  Vehicle Path Planner/1 -> Vehicle V2V Output/1
  Vehicle Sensors/1 -> V2V Communication Module/1
  Zero-Order Hold6/1 -> V_Network_Out/1

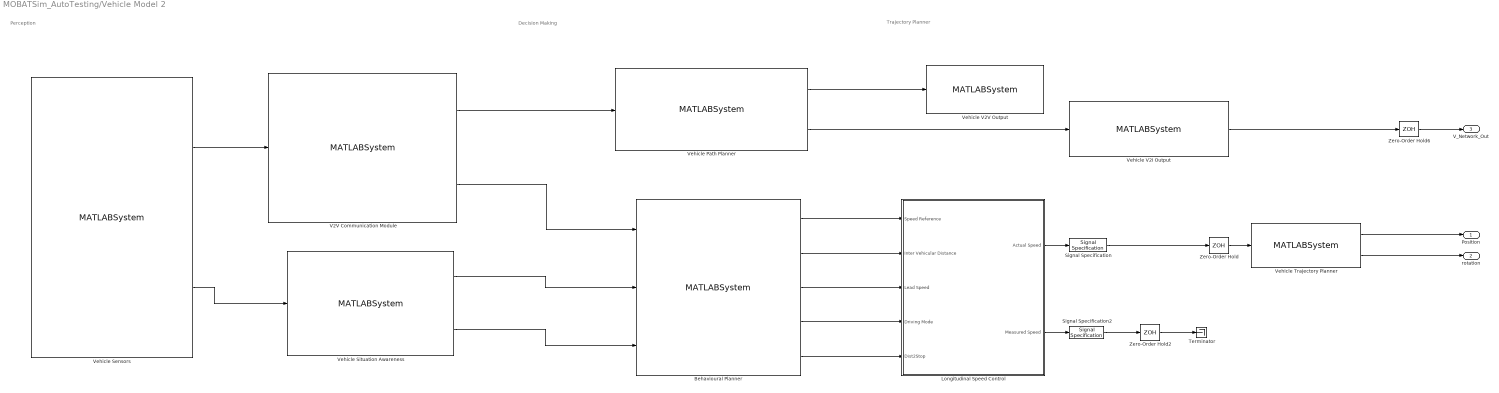
== system MOBATSim_AutoTesting/Vehicle Model 2 ==
  note: Trajectory Planner
  note: Perception
  note: Decision Making
  Behavioural Planner : MATLABSystem  System=VehicleDrivingMode  Vehicle_id=Vehicle_id  SimulateUsing=Interpreted execution
      mask Type: VehicleDrivingMode
      mask Display:
      | image('BehaviouralPlanner.png');
      | port_label('input',1,'LeaderSpeed');
      | port_label('input',2,'LeaderDistance');
      | port_label('input',3,'emergencyCase');
      | port_label('output',1,'SpeedReference');
      | port_label('output',2,'DistanceReference');
      | port_label('output',3,'LeadSpeed');
      | port_label('output',4,'DrivingMode');
      | port_label('output',5,'Dist2Stop');
  Longitudinal Speed Control : Subsystem
  Signal Specification : SignalSpecification  Dimensions=1
  Signal Specification2 : SignalSpecification  Dimensions=1
  Terminator : Terminator
  V2V Communication Module : MATLABSystem  System=VehicleCommunication_v2v  Vehicle_id=Vehicle_id  SimulateUsing=Interpreted execution
      mask Type: VehicleCommunication_v2v
      mask Display:
      | image('V2V.png');
      | port_label('input',1,'CommunicationID');
      | port_label('output',1,'OtherVehiclesFutureData');
      | port_label('output',2,'LeaderSpeed');
  Vehicle Path Planner : MATLABSystem  System=VehiclePathPlanner  Vehicle_id=Vehicle_id  SimulateUsing=Interpreted execution
      mask Type: VehiclePathPlanner
      mask Display:
      | image('PathPlanner.png');
      | port_label('input',1,'OtherVehiclesFutureData');
      | port_label('output',1,'FuturePlan');
      | port_label('output',2,'waypointReached');
  Vehicle Sensors : MATLABSystem  System=VehicleSensors  Vehicle_id=Vehicle_id  Tsample=Sim_Ts  OffsetTime=0  SimulateUsing=Interpreted execution
      mask Type: VehicleSensors
      mask Display:
      | image('sensor.png');
      | port_label('output',1,'V2VcommIDs');
      | port_label('output',2,'ObjectinFront');
  Vehicle Situation Awareness : MATLABSystem  System=VehicleSituationAwareness  Vehicle_id=Vehicle_id  SimulateUsing=Interpreted execution
      mask Type: VehicleSituationAwareness
      mask Display:
      | image('situationAwareness.png');
      | port_label('input',1,'FrontSensorData');
      | port_label('output',1,'leaderDistance');
      | port_label('output',2,'emergencyCase');
  Vehicle Trajectory Planner : MATLABSystem  System=VehicleKinematics  Vehicle_id=Vehicle_id  SimulateUsing=Interpreted execution
      mask Type: VehicleKinematics
      mask Display:
      | image('Vehicle.png');
      | port_label('input',1,'speed');
      | port_label('output',1,'position');
      | port_label('output',2,'rotation');
  Vehicle V2I Output : MATLABSystem  System=VehicleV2I_Out  Vehicle_id=Vehicle_id  SimulateUsing=Interpreted execution
      mask Type: VehicleV2I_Out
      mask Display:
      | image('V2I.png');
      | port_label('input',1,'waypointReached');
      | port_label('output',1,'V2Idata');
  Vehicle V2V Output : MATLABSystem  System=VehicleNetwork_Out  Vehicle_id=Vehicle_id  SimulateUsing=Interpreted execution
      mask Type: VehicleNetwork_Out
      mask Display:
      | image('V2V.png');
      | port_label('input',1,'FuturePlan');
  Zero-Order Hold : ZeroOrderHold  SampleTime=Sim_Ts
  Zero-Order Hold2 : ZeroOrderHold  SampleTime=Sim_Ts
  Zero-Order Hold6 : ZeroOrderHold  SampleTime=Sim_Ts
  Position : Outport  VectorParamsAs1DForOutWhenUnconnected=off
  rotation : Outport  Port=2  VectorParamsAs1DForOutWhenUnconnected=off
  V_Network_Out : Outport  Port=3  VectorParamsAs1DForOutWhenUnconnected=off
  wires:
  Vehicle Trajectory Planner/1 -> Position/1
  Vehicle Trajectory Planner/2 -> rotation/1
  Signal Specification/1 -> Zero-Order Hold/1
  Zero-Order Hold/1 -> Vehicle Trajectory Planner/1
  Signal Specification2/1 -> Zero-Order Hold2/1
  Longitudinal Speed Control/1(Actual Speed) -> Signal Specification/1
  Vehicle V2I Output/1 -> Zero-Order Hold6/1
  Longitudinal Speed Control/2(Measured Speed) -> Signal Specification2/1
  Zero-Order Hold2/1 -> Terminator/1
  Vehicle Sensors/2 -> Vehicle Situation Awareness/1
  Vehicle Situation Awareness/2 -> Behavioural Planner/3
  Vehicle Situation Awareness/1 -> Behavioural Planner/2
  V2V Communication Module/2 -> Behavioural Planner/1
  V2V Communication Module/1 -> Vehicle Path Planner/1
  Behavioural Planner/5 -> Longitudinal Speed Control/5(Dist2Stop)
  Behavioural Planner/4 -> Longitudinal Speed Control/4(Driving Mode)
  Behavioural Planner/3 -> Longitudinal Speed Control/3(Lead Speed)
  Behavioural Planner/2 -> Longitudinal Speed Control/2(Inter Vehicular Distance)
  Behavioural Planner/1 -> Longitudinal Speed Control/1(Speed Reference)
  Vehicle Path Planner/2 -> Vehicle V2I Output/1
  Vehicle Path Planner/1 -> Vehicle V2V Output/1
  Vehicle Sensors/1 -> V2V Communication Module/1
  Zero-Order Hold6/1 -> V_Network_Out/1

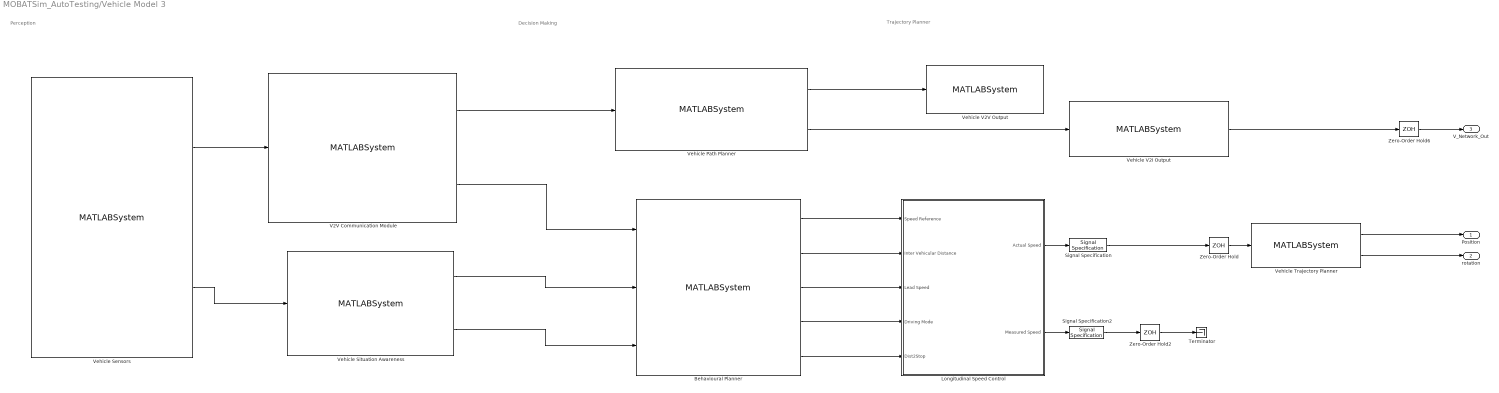
== system MOBATSim_AutoTesting/Vehicle Model 3 ==
  note: Trajectory Planner
  note: Perception
  note: Decision Making
  Behavioural Planner : MATLABSystem  System=VehicleDrivingMode  Vehicle_id=Vehicle_id  SimulateUsing=Interpreted execution
      mask Type: VehicleDrivingMode
      mask Display:
      | image('BehaviouralPlanner.png');
      | port_label('input',1,'LeaderSpeed');
      | port_label('input',2,'LeaderDistance');
      | port_label('input',3,'emergencyCase');
      | port_label('output',1,'SpeedReference');
      | port_label('output',2,'DistanceReference');
      | port_label('output',3,'LeadSpeed');
      | port_label('output',4,'DrivingMode');
      | port_label('output',5,'Dist2Stop');
  Longitudinal Speed Control : Subsystem
  Signal Specification : SignalSpecification  Dimensions=1
  Signal Specification2 : SignalSpecification  Dimensions=1
  Terminator : Terminator
  V2V Communication Module : MATLABSystem  System=VehicleCommunication_v2v  Vehicle_id=Vehicle_id  SimulateUsing=Interpreted execution
      mask Type: VehicleCommunication_v2v
      mask Display:
      | image('V2V.png');
      | port_label('input',1,'CommunicationID');
      | port_label('output',1,'OtherVehiclesFutureData');
      | port_label('output',2,'LeaderSpeed');
  Vehicle Path Planner : MATLABSystem  System=VehiclePathPlanner  Vehicle_id=Vehicle_id  SimulateUsing=Interpreted execution
      mask Type: VehiclePathPlanner
      mask Display:
      | image('PathPlanner.png');
      | port_label('input',1,'OtherVehiclesFutureData');
      | port_label('output',1,'FuturePlan');
      | port_label('output',2,'waypointReached');
  Vehicle Sensors : MATLABSystem  System=VehicleSensors  Vehicle_id=Vehicle_id  Tsample=Sim_Ts  OffsetTime=0  SimulateUsing=Interpreted execution
      mask Type: VehicleSensors
      mask Display:
      | image('sensor.png');
      | port_label('output',1,'V2VcommIDs');
      | port_label('output',2,'ObjectinFront');
  Vehicle Situation Awareness : MATLABSystem  System=VehicleSituationAwareness  Vehicle_id=Vehicle_id  SimulateUsing=Interpreted execution
      mask Type: VehicleSituationAwareness
      mask Display:
      | image('situationAwareness.png');
      | port_label('input',1,'FrontSensorData');
      | port_label('output',1,'leaderDistance');
      | port_label('output',2,'emergencyCase');
  Vehicle Trajectory Planner : MATLABSystem  System=VehicleKinematics  Vehicle_id=Vehicle_id  SimulateUsing=Interpreted execution
      mask Type: VehicleKinematics
      mask Display:
      | image('Vehicle.png');
      | port_label('input',1,'speed');
      | port_label('output',1,'position');
      | port_label('output',2,'rotation');
  Vehicle V2I Output : MATLABSystem  System=VehicleV2I_Out  Vehicle_id=Vehicle_id  SimulateUsing=Interpreted execution
      mask Type: VehicleV2I_Out
      mask Display:
      | image('V2I.png');
      | port_label('input',1,'waypointReached');
      | port_label('output',1,'V2Idata');
  Vehicle V2V Output : MATLABSystem  System=VehicleNetwork_Out  Vehicle_id=Vehicle_id  SimulateUsing=Interpreted execution
      mask Type: VehicleNetwork_Out
      mask Display:
      | image('V2V.png');
      | port_label('input',1,'FuturePlan');
  Zero-Order Hold : ZeroOrderHold  SampleTime=Sim_Ts
  Zero-Order Hold2 : ZeroOrderHold  SampleTime=Sim_Ts
  Zero-Order Hold6 : ZeroOrderHold  SampleTime=Sim_Ts
  Position : Outport  VectorParamsAs1DForOutWhenUnconnected=off
  rotation : Outport  Port=2  VectorParamsAs1DForOutWhenUnconnected=off
  V_Network_Out : Outport  Port=3  VectorParamsAs1DForOutWhenUnconnected=off
  wires:
  Vehicle Trajectory Planner/1 -> Position/1
  Vehicle Trajectory Planner/2 -> rotation/1
  Signal Specification/1 -> Zero-Order Hold/1
  Zero-Order Hold/1 -> Vehicle Trajectory Planner/1
  Signal Specification2/1 -> Zero-Order Hold2/1
  Longitudinal Speed Control/1(Actual Speed) -> Signal Specification/1
  Vehicle V2I Output/1 -> Zero-Order Hold6/1
  Longitudinal Speed Control/2(Measured Speed) -> Signal Specification2/1
  Zero-Order Hold2/1 -> Terminator/1
  Vehicle Sensors/2 -> Vehicle Situation Awareness/1
  Vehicle Situation Awareness/2 -> Behavioural Planner/3
  Vehicle Situation Awareness/1 -> Behavioural Planner/2
  V2V Communication Module/2 -> Behavioural Planner/1
  V2V Communication Module/1 -> Vehicle Path Planner/1
  Behavioural Planner/5 -> Longitudinal Speed Control/5(Dist2Stop)
  Behavioural Planner/4 -> Longitudinal Speed Control/4(Driving Mode)
  Behavioural Planner/3 -> Longitudinal Speed Control/3(Lead Speed)
  Behavioural Planner/2 -> Longitudinal Speed Control/2(Inter Vehicular Distance)
  Behavioural Planner/1 -> Longitudinal Speed Control/1(Speed Reference)
  Vehicle Path Planner/2 -> Vehicle V2I Output/1
  Vehicle Path Planner/1 -> Vehicle V2V Output/1
  Vehicle Sensors/1 -> V2V Communication Module/1
  Zero-Order Hold6/1 -> V_Network_Out/1

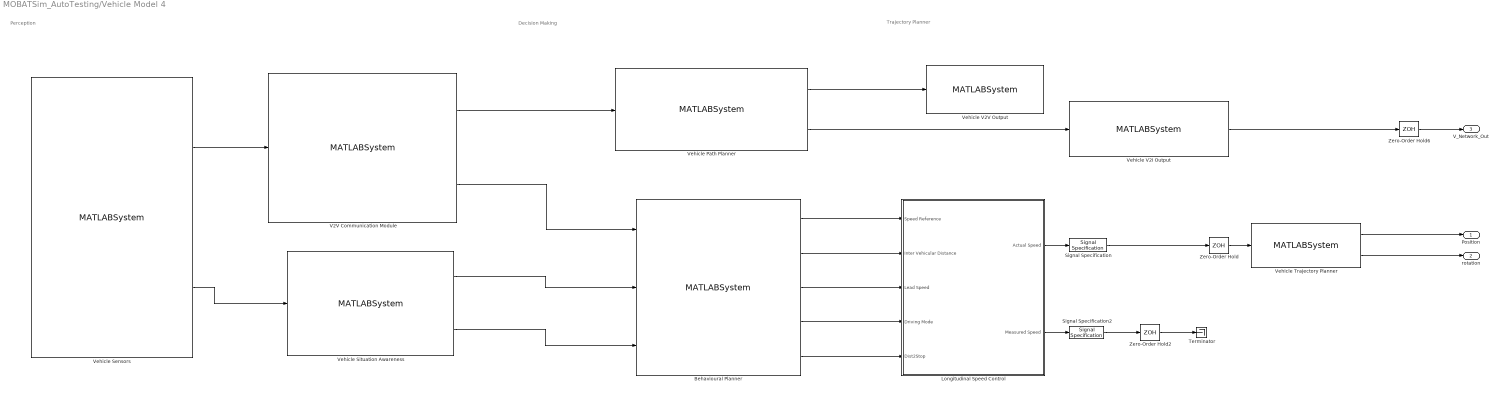
== system MOBATSim_AutoTesting/Vehicle Model 4 ==
  note: Trajectory Planner
  note: Perception
  note: Decision Making
  Behavioural Planner : MATLABSystem  System=VehicleDrivingMode  Vehicle_id=Vehicle_id  SimulateUsing=Interpreted execution
      mask Type: VehicleDrivingMode
      mask Display:
      | image('BehaviouralPlanner.png');
      | port_label('input',1,'LeaderSpeed');
      | port_label('input',2,'LeaderDistance');
      | port_label('input',3,'emergencyCase');
      | port_label('output',1,'SpeedReference');
      | port_label('output',2,'DistanceReference');
      | port_label('output',3,'LeadSpeed');
      | port_label('output',4,'DrivingMode');
      | port_label('output',5,'Dist2Stop');
  Longitudinal Speed Control : Subsystem
  Signal Specification : SignalSpecification  Dimensions=1
  Signal Specification2 : SignalSpecification  Dimensions=1
  Terminator : Terminator
  V2V Communication Module : MATLABSystem  System=VehicleCommunication_v2v  Vehicle_id=Vehicle_id  SimulateUsing=Interpreted execution
      mask Type: VehicleCommunication_v2v
      mask Display:
      | image('V2V.png');
      | port_label('input',1,'CommunicationID');
      | port_label('output',1,'OtherVehiclesFutureData');
      | port_label('output',2,'LeaderSpeed');
  Vehicle Path Planner : MATLABSystem  System=VehiclePathPlanner  Vehicle_id=Vehicle_id  SimulateUsing=Interpreted execution
      mask Type: VehiclePathPlanner
      mask Display:
      | image('PathPlanner.png');
      | port_label('input',1,'OtherVehiclesFutureData');
      | port_label('output',1,'FuturePlan');
      | port_label('output',2,'waypointReached');
  Vehicle Sensors : MATLABSystem  System=VehicleSensors  Vehicle_id=Vehicle_id  Tsample=Sim_Ts  OffsetTime=0  SimulateUsing=Interpreted execution
      mask Type: VehicleSensors
      mask Display:
      | image('sensor.png');
      | port_label('output',1,'V2VcommIDs');
      | port_label('output',2,'ObjectinFront');
  Vehicle Situation Awareness : MATLABSystem  System=VehicleSituationAwareness  Vehicle_id=Vehicle_id  SimulateUsing=Interpreted execution
      mask Type: VehicleSituationAwareness
      mask Display:
      | image('situationAwareness.png');
      | port_label('input',1,'FrontSensorData');
      | port_label('output',1,'leaderDistance');
      | port_label('output',2,'emergencyCase');
  Vehicle Trajectory Planner : MATLABSystem  System=VehicleKinematics  Vehicle_id=Vehicle_id  SimulateUsing=Interpreted execution
      mask Type: VehicleKinematics
      mask Display:
      | image('Vehicle.png');
      | port_label('input',1,'speed');
      | port_label('output',1,'position');
      | port_label('output',2,'rotation');
  Vehicle V2I Output : MATLABSystem  System=VehicleV2I_Out  Vehicle_id=Vehicle_id  SimulateUsing=Interpreted execution
      mask Type: VehicleV2I_Out
      mask Display:
      | image('V2I.png');
      | port_label('input',1,'waypointReached');
      | port_label('output',1,'V2Idata');
  Vehicle V2V Output : MATLABSystem  System=VehicleNetwork_Out  Vehicle_id=Vehicle_id  SimulateUsing=Interpreted execution
      mask Type: VehicleNetwork_Out
      mask Display:
      | image('V2V.png');
      | port_label('input',1,'FuturePlan');
  Zero-Order Hold : ZeroOrderHold  SampleTime=Sim_Ts
  Zero-Order Hold2 : ZeroOrderHold  SampleTime=Sim_Ts
  Zero-Order Hold6 : ZeroOrderHold  SampleTime=Sim_Ts
  Position : Outport  VectorParamsAs1DForOutWhenUnconnected=off
  rotation : Outport  Port=2  VectorParamsAs1DForOutWhenUnconnected=off
  V_Network_Out : Outport  Port=3  VectorParamsAs1DForOutWhenUnconnected=off
  wires:
  Vehicle Trajectory Planner/1 -> Position/1
  Vehicle Trajectory Planner/2 -> rotation/1
  Signal Specification/1 -> Zero-Order Hold/1
  Zero-Order Hold/1 -> Vehicle Trajectory Planner/1
  Signal Specification2/1 -> Zero-Order Hold2/1
  Longitudinal Speed Control/1(Actual Speed) -> Signal Specification/1
  Vehicle V2I Output/1 -> Zero-Order Hold6/1
  Longitudinal Speed Control/2(Measured Speed) -> Signal Specification2/1
  Zero-Order Hold2/1 -> Terminator/1
  Vehicle Sensors/2 -> Vehicle Situation Awareness/1
  Vehicle Situation Awareness/2 -> Behavioural Planner/3
  Vehicle Situation Awareness/1 -> Behavioural Planner/2
  V2V Communication Module/2 -> Behavioural Planner/1
  V2V Communication Module/1 -> Vehicle Path Planner/1
  Behavioural Planner/5 -> Longitudinal Speed Control/5(Dist2Stop)
  Behavioural Planner/4 -> Longitudinal Speed Control/4(Driving Mode)
  Behavioural Planner/3 -> Longitudinal Speed Control/3(Lead Speed)
  Behavioural Planner/2 -> Longitudinal Speed Control/2(Inter Vehicular Distance)
  Behavioural Planner/1 -> Longitudinal Speed Control/1(Speed Reference)
  Vehicle Path Planner/2 -> Vehicle V2I Output/1
  Vehicle Path Planner/1 -> Vehicle V2V Output/1
  Vehicle Sensors/1 -> V2V Communication Module/1
  Zero-Order Hold6/1 -> V_Network_Out/1
